simulink library "dlbsBlockGain"  (R2025b)
settings: Solver=VariableStepAuto  StartTime=0.0  StopTime=10.0  RelTol=1e-3
libraries: dlbsBlockExtractGradientGF x1, dlbsBlockInsertGradientGF x1
settings Model: Creator=lt6037  LastModifiedBy=lt6037

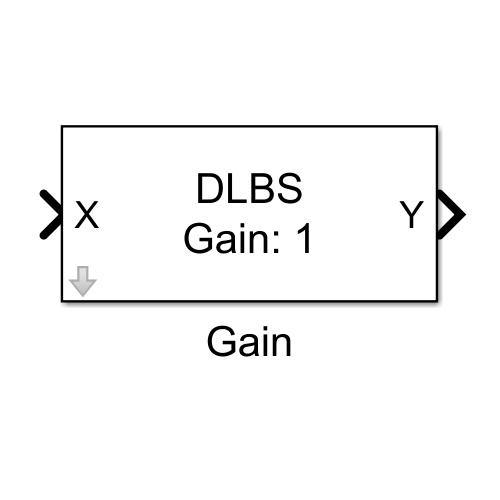
[thumbnail: Simulink's stored preview of the top-level diagram]
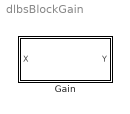
== system dlbsBlockGain ==
  Gain : Subsystem  mask{Gain=1}
      mask prompts: Gain "Simulink:blkprm_prompts:GainGain"
      mask help: Scales the input tensor by a gain parameter. The operation is applied element-wise across all tensor elements.
      mask Help: web("dlbsHelpBlockGain.html")
      mask TypeOptions Gain: Gain/Gain | Gain1/Gain
      mask DialogControl Gain Prompt: Gain:
      mask Display: fprintf("DLBS\nGain: %s",get(gcbh).Gain)

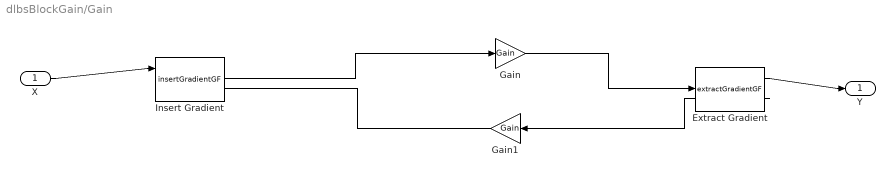
== system dlbsBlockGain/Gain ==
  X : Inport
  Extract Gradient : dlbsBlockExtractGradientGF/extractGradientGF
  Gain : Gain  Gain=Gain
  Gain1 : Gain  Gain=Gain
  Insert Gradient : dlbsBlockInsertGradientGF/insertGradientGF
  Y : Outport
  wires:
  Extract Gradient/1 -> Y/1
  X/1 -> Insert Gradient/1
  Extract Gradient/2 -> Gain1/1
  Gain/1 -> Extract Gradient/1
  Insert Gradient/1 -> Gain/1
  Gain1/1 -> Insert Gradient/2
